simulink model "sample06_position"  (R2023a)
settings: Solver=ode1  StartTime=0.0  StopTime=inf  FixedStep=0.005  RelTol=1e-3  EnableMultiTasking=on
libraries: arduinolib x8, simulink x4
settings Model: ExtModeTrigDuration=2  Creator=kawata  LastModifiedBy=kawata
settings SolverCC: AutoInsertRateTranBlk=on
settings DataIOCC: ReturnWorkspaceOutputs=off
settings OptimizationCC: EnhancedBackFolding=on  PassReuseOutputArgsAs=Individual arguments  ZeroExternalMemoryAtStartup=off  ZeroInternalMemoryAtStartup=off  MaxStackSize=64  OptimizeBlockOrder=speed  DifferentSizesBufferReuse=on  OptimizationCustomize=off  EfficientTunableParamExpr=on
settings DebuggingCC: ParameterTunabilityLossMsg=error
settings HardwareCC: ProdBitPerPointer=32  ProdBitPerSizeT=32  ProdBitPerPtrDiffT=32  ProdLargestAtomicInteger=Long  ProdLargestAtomicFloat=Double  ProdWordSize=32  ProdHWDeviceType=ARM Compatible->ARM Cortex  UseEmbeddedCoderFeatures=off  UseSimulinkCoderFeatures=off
settings SFSimCC: MATLABDynamicMemAlloc=off
settings RTWCC: Description=Embedded Coder  SystemTargetFile=ert.tlc  HardwareBoard=ESP32-WROOM(Arduino Compatible)  TLCOptions="-aInlineSetEventsForThisBaseRateFcn=TLC_FALSE -aSuppressMultiTaskScheduler=TLC_FALSE  -aRateBasedStepFcn=0"  TemplateMakefile=ert_default_tmf  Toolchain=ESP32  BuildConfiguration=Faster Runs  GPUComputeCapability=5.0
settings CodeAppCC: ForceParamTrailComments=on  IgnoreCustomStorageClasses=off  OperatorAnnotations=on  SimulinkDataObjDesc=on  SFDataObjDesc=on  InsertBlockDesc=on
settings ERTTargetCC: SupportContinuousTime=on  SupportNonInlinedSFcns=on  SupportVariableSizeSignals=on  ExtModeTransport=3  ExtModeStaticAlloc=on  ExtModeAutomaticAllocSize=off  ExtModeStaticAllocSize=65536  ExtModeMexFile=ext_xcp  ExtModeIntrfLevel=Level2 - Open

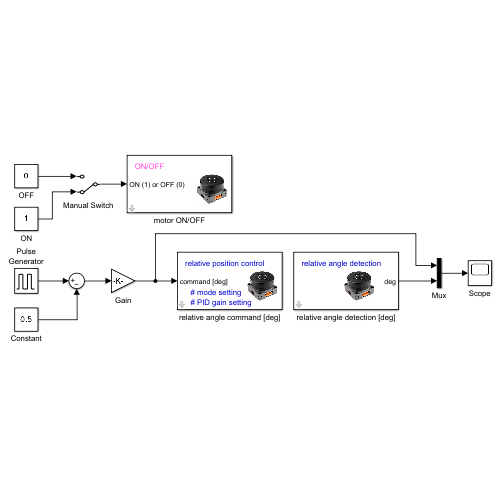
[thumbnail: Simulink's stored preview of the top-level diagram]
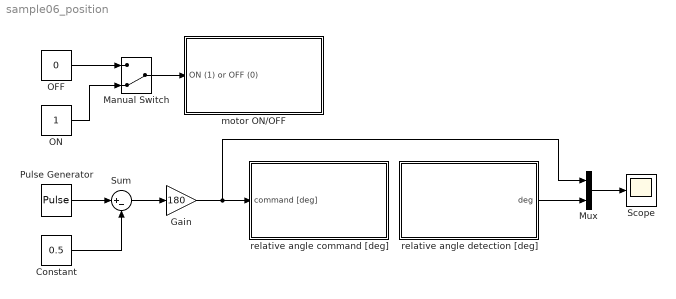
== system sample06_position ==
  Constant : Constant  Value=0.5
  Gain : Gain  Gain=180
  Manual Switch : ManualSwitch  CurrentSetting=0
  Mux : Mux  Inputs=2
  OFF : Constant  Value=0
  ON : Constant
  Pulse Generator : DiscretePulseGenerator  PulseType=Time based  Period=4  PulseWidth=50  PhaseDelay=1
  Scope : Scope
  Sum : Sum  Inputs=|+-
  motor ON/OFF : Subsystem  mask{I2CAddress=0x64}
      mask prompts: I2CAddress "I2C Address"
      mask help:
      | 0: motor off
      | 1: motor on
      mask DialogControl ParameterGroupVar Prompt: パラメーター
      mask Display:
      | image('roller485.png', [55,10,75,56]);
      | color('magenta');
      | text(10, 60, 'ON/OFF');
  relative angle command [deg] : Subsystem  mask(relative angle command [deg]){I2CAddress=0x64, sample_time=0.005, set_time=0, position_P=15, position_I=0.000003, position_D=400}
      mask prompts: I2CAddress "I2C Address"; sample_time "Sample Time"; set_time "Set Time"; position_P "P"; position_I "I"; position_D "D"
      mask help:
      | position mode
      | ---------------------------------
      | default value (PID gain of position controller)
      |  P: 15
      |  I: 0.000003
      |  D: 400
      | ---------------------------------
      | If t ≤ set_time, then PID gain can be set.
      mask DialogControl ParameterGroupVar Prompt: パラメーター
      mask Display:
      | image('roller485.png', [55,10,75,56]);
      | color('blue');
      | text(10, 60, 'relative position control');
      | text(17, 22, '# mode setting');
      | text(17, 10, '# PID gain setting');
  relative angle detection [deg] : Subsystem  mask{I2CAddress=0x64, sample_time=0.005}
      mask prompts: I2CAddress "I2C Address"; sample_time "Sample Time"
      mask DialogControl ParameterGroupVar Prompt: パラメーター
      mask Display:
      | image('roller485.png', [30,10,75,56]);
      | color('blue');
      | text(10, 60, 'relative angle detection');
  wires:
  Manual Switch/1 -> motor ON/OFF/1(ON (1) or OFF (0))
  OFF/1 -> Manual Switch/1
  ON/1 -> Manual Switch/2
  Gain/1 -> relative angle command [deg]/1(command [deg]), Mux/1
  Sum/1 -> Gain/1
  Constant/1 -> Sum/2
  Pulse Generator/1 -> Sum/1
  relative angle detection [deg]/1(deg) -> Mux/2
  Mux/1 -> Scope/1

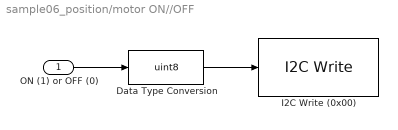
== system sample06_position/motor ON//OFF ==
  ON (1) or OFF (0) : Inport
  Data Type Conversion : DataTypeConversion  OutDataTypeStr=uint8  SaturateOnIntegerOverflow=off  RndMeth=Floor
  I2C Write (0x00) : arduinolib/I2C Write  I2CModule=0  Mode=Master  SlaveAddress=I2CAddress  SlaveByteOrder=BigEndian  Direction=Transmitter  RegisterAddressMode=on  RegisterAddress=0x00  SlaveDataType=uint8  DataLength=1  NoAck=off  RepeatedStart=off  OutputStatus=off  blockPlatform=ARDUINO
  wires:
  Data Type Conversion/1 -> I2C Write (0x00)/1
  ON (1) or OFF (0)/1 -> Data Type Conversion/1

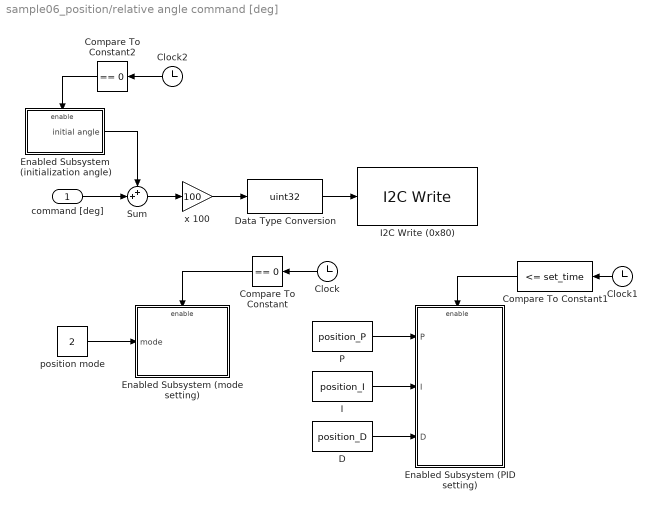
== system sample06_position/relative angle command [deg] ==
  command [deg] : Inport
  "Clock " : Clock
  Clock1 : Clock
  Clock2 : Clock
  Compare To Constant : simulink/Logic and Bit Operations/Compare To Constant  relop===  const=0  OutDataTypeStr=boolean
  Compare To Constant1 : simulink/Logic and Bit Operations/Compare To Constant  relop=<=  const=set_time  OutDataTypeStr=boolean
  Compare To Constant2 : simulink/Logic and Bit Operations/Compare To Constant  relop===  const=0  OutDataTypeStr=boolean
  D : Constant  Value=position_D
  Data Type Conversion : DataTypeConversion  OutDataTypeStr=uint32  SaturateOnIntegerOverflow=off  RndMeth=Floor
  Enabled Subsystem (PID setting) : Subsystem  TreatAsAtomicUnit=on
  Enabled Subsystem (initialization angle) : Subsystem  TreatAsAtomicUnit=on
  Enabled Subsystem (mode setting) : Subsystem  TreatAsAtomicUnit=on
  I : Constant  Value=position_I
  I2C Write (0x80) : arduinolib/I2C Write  I2CModule=0  Mode=Master  SlaveAddress=I2CAddress  SlaveByteOrder=LittleEndian  Direction=Transmitter  RegisterAddressMode=on  RegisterAddress=0x80  SlaveDataType=uint8  DataLength=1  NoAck=off  RepeatedStart=off  OutputStatus=off  blockPlatform=ARDUINO
  P : Constant  Value=position_P
  Sum : Sum  Inputs=++|
  position mode : Constant  Value=2
  x 100 : Gain  Gain=100
  wires:
  Clock1/1 -> Compare To Constant1/1
  x 100/1 -> Data Type Conversion/1
  D/1 -> Enabled Subsystem (PID setting)/3(D)
  Sum/1 -> x 100/1
  Enabled Subsystem (initialization angle)/1(initial angle) -> Sum/1
  command [deg]/1 -> Sum/2
  Clock2/1 -> Compare To Constant2/1
  Compare To Constant2/1 -> Enabled Subsystem (initialization angle)/Enable
  Data Type Conversion/1 -> I2C Write (0x80)/1
  I/1 -> Enabled Subsystem (PID setting)/2(I)
  P/1 -> Enabled Subsystem (PID setting)/1(P)
  position mode/1 -> Enabled Subsystem (mode setting)/1(mode)
  Compare To Constant1/1 -> Enabled Subsystem (PID setting)/Enable
  Compare To Constant/1 -> Enabled Subsystem (mode setting)/Enable
  "Clock "/1 -> Compare To Constant/1

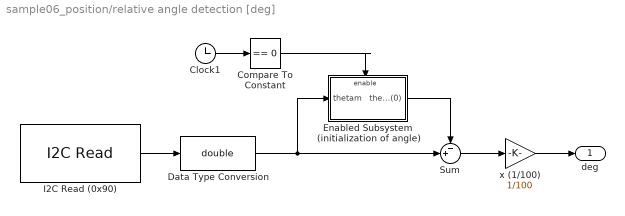
== system sample06_position/relative angle detection [deg] ==
  Clock1 : Clock
  Compare To Constant : simulink/Logic and Bit Operations/Compare To Constant  relop===  const=0  OutDataTypeStr=boolean
  Data Type Conversion : DataTypeConversion  OutDataTypeStr=double  SaturateOnIntegerOverflow=off  RndMeth=Floor
  Enabled Subsystem (initialization of angle) : Subsystem  TreatAsAtomicUnit=on
  I2C Read (0x90) : arduinolib/I2C Read  I2CModule=0  Mode=Master  SlaveAddress=0x64  SlaveByteOrder=LittleEndian  Direction=Receiver  RegisterAddressMode=on  RegisterAddress=0x90  SlaveDataType=int32  DataLength=1  NoAck=off  RepeatedStart=off  OutputStatus=off  blockPlatform=ARDUINO  SampleTime=sample_time
  Sum : Sum  Inputs=-+|
  x (1/100) : Gain  Gain=1/100
  deg : Outport
  wires:
  I2C Read (0x90)/1 -> Data Type Conversion/1
  x (1/100)/1 -> deg/1
  Clock1/1 -> Compare To Constant/1
  Compare To Constant/1 -> Enabled Subsystem (initialization of angle)/Enable
  Data Type Conversion/1 -> Enabled Subsystem (initialization of angle)/1(thetam), Sum/2
  Enabled Subsystem (initialization of angle)/1(thetam(0)) -> Sum/1
  Sum/1 -> x (1/100)/1

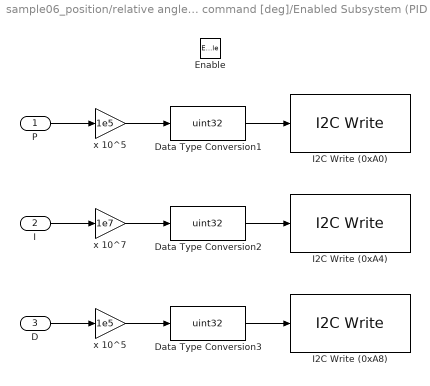
== system sample06_position/relative angle command [deg]/Enabled Subsystem (PID setting) ==
  P : Inport
  I : Inport  Port=2
  D : Inport  Port=3
  Enable : EnablePort
  " x 10^5 " : Gain  Gain=1e5
  Data Type Conversion1 : DataTypeConversion  OutDataTypeStr=uint32  SaturateOnIntegerOverflow=off  RndMeth=Floor
  Data Type Conversion2 : DataTypeConversion  OutDataTypeStr=uint32  SaturateOnIntegerOverflow=off  RndMeth=Floor
  Data Type Conversion3 : DataTypeConversion  OutDataTypeStr=uint32  SaturateOnIntegerOverflow=off  RndMeth=Floor
  I2C Write (0xA0) : arduinolib/I2C Write  I2CModule=0  Mode=Master  SlaveAddress=I2CAddress  SlaveByteOrder=LittleEndian  Direction=Transmitter  RegisterAddressMode=on  RegisterAddress=0xA0  SlaveDataType=uint8  DataLength=1  NoAck=off  RepeatedStart=off  OutputStatus=off  blockPlatform=ARDUINO
  I2C Write (0xA4) : arduinolib/I2C Write  I2CModule=0  Mode=Master  SlaveAddress=I2CAddress  SlaveByteOrder=LittleEndian  Direction=Transmitter  RegisterAddressMode=on  RegisterAddress=0xA4  SlaveDataType=uint8  DataLength=1  NoAck=off  RepeatedStart=off  OutputStatus=off  blockPlatform=ARDUINO
  I2C Write (0xA8) : arduinolib/I2C Write  I2CModule=0  Mode=Master  SlaveAddress=I2CAddress  SlaveByteOrder=LittleEndian  Direction=Transmitter  RegisterAddressMode=on  RegisterAddress=0xA8  SlaveDataType=uint8  DataLength=1  NoAck=off  RepeatedStart=off  OutputStatus=off  blockPlatform=ARDUINO
  x 10^5 : Gain  Gain=1e5
  x 10^7 : Gain  Gain=1e7
  wires:
  " x 10^5 "/1 -> Data Type Conversion3/1
  x 10^7/1 -> Data Type Conversion2/1
  x 10^5/1 -> Data Type Conversion1/1
  Data Type Conversion1/1 -> I2C Write (0xA0)/1
  Data Type Conversion3/1 -> I2C Write (0xA8)/1
  Data Type Conversion2/1 -> I2C Write (0xA4)/1
  D/1 -> " x 10^5 "/1
  I/1 -> x 10^7/1
  P/1 -> x 10^5/1

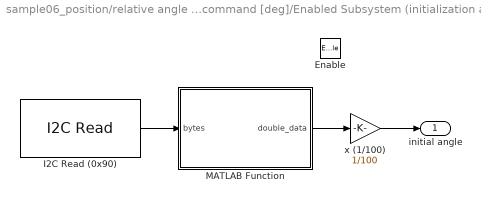
== system sample06_position/relative angle command [deg]/Enabled Subsystem (initialization angle) ==
  Enable : EnablePort
  I2C Read (0x90) : arduinolib/I2C Read  I2CModule=0  Mode=Master  SlaveAddress=0x64  SlaveByteOrder=BigEndian  Direction=Receiver  RegisterAddressMode=on  RegisterAddress=0x90  SlaveDataType=uint8  DataLength=4  NoAck=off  RepeatedStart=off  OutputStatus=off  blockPlatform=ARDUINO  SampleTime=sample_time
  MATLAB Function : MATLAB Function  TreatAsAtomicUnit=on
  x (1/100) : Gain  Gain=1/100
  initial angle : Outport
  wires:
  x (1/100)/1 -> initial angle/1
  I2C Read (0x90)/1 -> MATLAB Function/1(bytes)
  MATLAB Function/1(double_data) -> x (1/100)/1

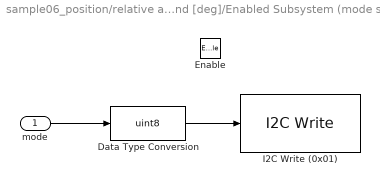
== system sample06_position/relative angle command [deg]/Enabled Subsystem (mode setting) ==
  mode : Inport
  Enable : EnablePort
  Data Type Conversion : DataTypeConversion  OutDataTypeStr=uint8  SaturateOnIntegerOverflow=off  RndMeth=Floor
  I2C Write (0x01) : arduinolib/I2C Write  I2CModule=0  Mode=Master  SlaveAddress=I2CAddress  SlaveByteOrder=BigEndian  Direction=Transmitter  RegisterAddressMode=on  RegisterAddress=0x01  SlaveDataType=uint8  DataLength=1  NoAck=off  RepeatedStart=off  OutputStatus=off  blockPlatform=ARDUINO
  wires:
  Data Type Conversion/1 -> I2C Write (0x01)/1
  mode/1 -> Data Type Conversion/1

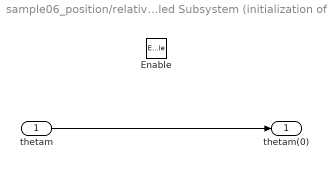
== system sample06_position/relative angle detection [deg]/Enabled Subsystem (initialization of angle) ==
  thetam : Inport
  Enable : EnablePort
  thetam(0) : Outport
  wires:
  thetam/1 -> thetam(0)/1

== matlab function sample06_position/relative angle command [deg]/Enabled Subsystem (initialization angle)/MATLAB Function ==
  data: bytes input; double_data output
function double_data = bytes_uint8_to_double(bytes)

double_data    = zeros(1, 1, 'double');    % 明示的に型とサイズを宣言
unsigned_int   = typecast(uint8(bytes), 'uint32');
signed_int     = typecast(unsigned_int, 'int32');
double_data(1) = double(signed_int);       % サイズを明示
